simulink model "Hw1_ME8352sim"  (R2020b)
settings: Solver=VariableStepAuto  StartTime=0.0  StopTime=t_sim  FixedStep=1e-3  RelTol=1e-3
values from neighbouring files (symbols this model uses):
  c = 1    [Hw1_ME8352.m]
  k = 1    [Hw1_ME8352.m]
  m = 1    [Hw1_ME8352.m]
  step_val = step_array(i)    [Hw1_ME8352.m]
  vdot0 = 0    [Hw1_ME8352.m]
  x_0 = x0_array(i)    [Hw1_ME8352.m]
  x_dot0 = xdot0_array(ii)    [Hw1_ME8352.m]
settings Model: Creator=dempseca  LastModifiedBy=dempseca

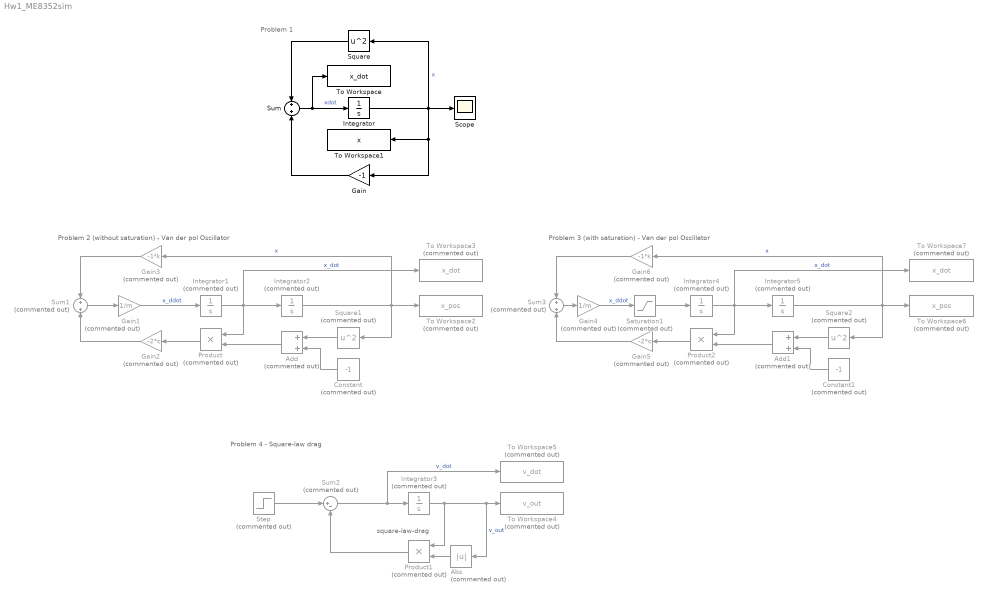
== system Hw1_ME8352sim ==
  note: Problem 4 - Square-law drag
  note: square-law-drag
  note: Problem 2 (without saturation) - Van der pol Oscillator
  note: Problem 1
  note: Problem 3 (with saturation) - Van der pol Oscillator
  Abs : Abs  Commented=on
  Add : Sum  Commented=on
  Add1 : Sum  Commented=on
  Constant : Constant  Commented=on  Value=-1
  Constant1 : Constant  Commented=on  Value=-1
  Gain : Gain  Gain=-1
  Gain1 : Gain  Commented=on  Gain=1/m
  Gain2 : Gain  Commented=on  Gain=-2*c
  Gain3 : Gain  Commented=on  Gain=-1*k
  Gain4 : Gain  Commented=on  Gain=1/m
  Gain5 : Gain  Commented=on  Gain=-2*c
  Gain6 : Gain  Commented=on  Gain=-1*k
  Integrator : Integrator  InitialCondition=x_dot0
  Integrator1 : Integrator  Commented=on  InitialCondition=x_dot0
  Integrator2 : Integrator  Commented=on  InitialCondition=x_0
  Integrator3 : Integrator  Commented=on  InitialCondition=vdot0
  Integrator4 : Integrator  Commented=on  InitialCondition=x_dot0
  Integrator5 : Integrator  Commented=on  InitialCondition=x_0
  Product : Product  Commented=on
  Product1 : Product  Commented=on
  Product2 : Product  Commented=on
  Saturation1 : Saturate  Commented=on  UpperLimit=1.5  LowerLimit=-1.5
  Scope : Scope
  Square : Math  Operator=square  SaturateOnIntegerOverflow=on
  Square1 : Math  Commented=on  Operator=square  SaturateOnIntegerOverflow=on
  Square2 : Math  Commented=on  Operator=square  SaturateOnIntegerOverflow=on
  Step : Step  Commented=on  Time=0  After=step_val  SampleTime=0
  Sum : Sum
  Sum1 : Sum  Commented=on
  Sum2 : Sum  Commented=on  Inputs=|+-
  Sum3 : Sum  Commented=on
  To Workspace : ToWorkspace  VariableName=x_dot  SaveFormat=Timeseries  SampleTime=-1
  To Workspace1 : ToWorkspace  VariableName=x  SaveFormat=Timeseries  SampleTime=-1
  To Workspace2 : ToWorkspace  Commented=on  VariableName=x_pos  SaveFormat=Timeseries  SampleTime=-1
  To Workspace3 : ToWorkspace  Commented=on  VariableName=x_dot  SaveFormat=Timeseries  SampleTime=-1
  To Workspace4 : ToWorkspace  Commented=on  VariableName=v_out  SaveFormat=Timeseries  SampleTime=-1
  To Workspace5 : ToWorkspace  Commented=on  VariableName=v_dot  SaveFormat=Timeseries  SampleTime=-1
  To Workspace6 : ToWorkspace  Commented=on  VariableName=x_pos  SaveFormat=Timeseries  SampleTime=-1
  To Workspace7 : ToWorkspace  Commented=on  VariableName=x_dot  SaveFormat=Timeseries  SampleTime=-1
  wires:
  Integrator/1 -> To Workspace1/1, Gain/1, Square/1, Scope/1  "x"
  Sum/1 -> To Workspace/1, Integrator/1  "xdot"
  Gain/1 -> Sum/2
  Square/1 -> Sum/1
  Integrator1/1 -> To Workspace3/1, Product/1, Integrator2/1  "x_dot"
  Gain1/1 -> Integrator1/1  "x_ddot"
  Integrator2/1 -> Gain3/1, Square1/1, To Workspace2/1  "x"
  Sum1/1 -> Gain1/1
  Square1/1 -> Add/1
  Constant/1 -> Add/2
  Add/1 -> Product/2
  Product/1 -> Gain2/1
  Gain2/1 -> Sum1/2
  Gain3/1 -> Sum1/1
  Integrator3/1 -> Product1/1, Abs/1, To Workspace4/1  "v_out"
  Sum2/1 -> To Workspace5/1, Integrator3/1  "v_dot"
  Step/1 -> Sum2/1
  Abs/1 -> Product1/2
  Product1/1 -> Sum2/2
  Integrator5/1 -> Gain6/1, Square2/1, To Workspace6/1  "x"
  Gain4/1 -> Saturation1/1  "x_ddot"
  Square2/1 -> Add1/1
  Sum3/1 -> Gain4/1
  Gain6/1 -> Sum3/1
  Product2/1 -> Gain5/1
  Integrator4/1 -> To Workspace7/1, Product2/1, Integrator5/1  "x_dot"
  Gain5/1 -> Sum3/2
  Constant1/1 -> Add1/2
  Add1/1 -> Product2/2
  Saturation1/1 -> Integrator4/1
